simulink model "Main"  (R2022b)
settings: Solver=VariableStepAuto  StartTime=0.0  StopTime=3.0  RelTol=1e-3
undefined symbols (not defined in the file): a, dc, I, K, L, m
settings Model: Creator=pagli  LastModifiedBy=pagli
settings SolverCC: ZeroCrossControl=DisableAll

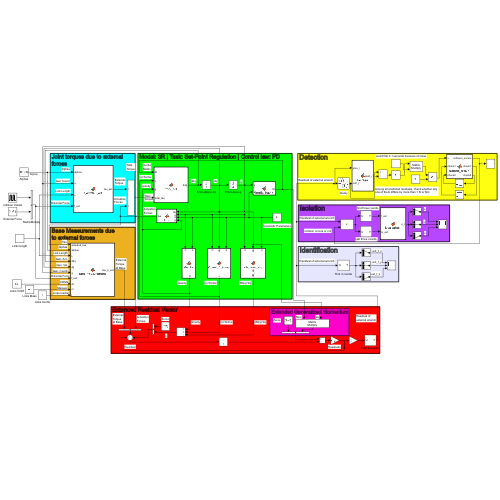
[thumbnail: Simulink's stored preview of the top-level diagram]
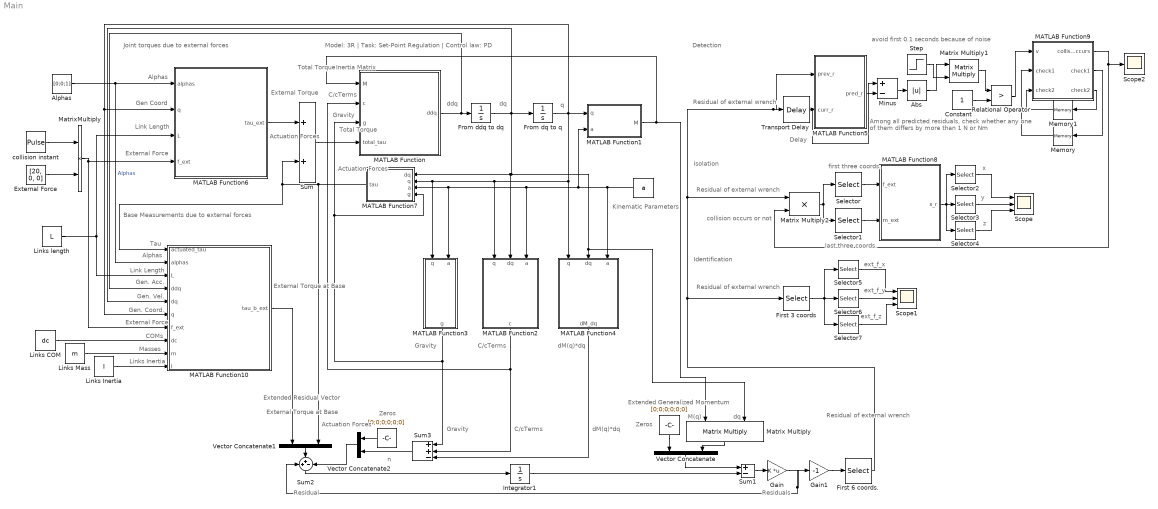
== system Main ==
  note: ext_f_x
  note: z
  note: y
  note: x
  note: Among all predicted residuals, check whether any
      | one of them differs by more than 1 N or Nm
  note: avoid first 0.1 seconds because of noise
  note: Delay
  note: first three coords.
  note: collision occurs or not
  note: Extended Generalized Momentum
  note: Identification
  note: Tau
  note: Alphas
  note: Isolation
  note: Detection
  note: n
  note: Residual
  note: External
      | Torque
      | at Base
  note: Links Inertia
  note: Masses
  note: COMs
  note: Gen. Coord.
  note: Gen. Vel.
  note: Gen. Acc.
  note: dM(q)*dq
  note: Kinematic Parameters
  note: q
  note: dq
  note: ddq
  note: Actuation
      | Forces
  note: Gravity
  note: C/cTerms
  note: Inertia
      | Matrix
  note: External
      | Torque
  note: External Force
  note: Link Length
  note: Gen Coord
  note: Alphas
  note: Zeros
  note: M(q)
  note: dq
  note: Joint torques due to external
      | forces
  note: Base Measurements due
      | to external forces
  note: Model: 3R | Task: Set-Point Regulation | Control law: PD
  note: Extended Residual Vector
  note: Zeros
  note: Total
      | Torque
  note: Gravity
  note: C/cTerms
  note: Link Length
  note: External Force
  note: External
      | Torque
      | at Base
  note: Actuation
      | Forces
  note: Gravity
  note: C/cTerms
  note: dM(q)*dq
  note: Residuals
  note: Residual of external wrench
  note: Residual of external wrench
  note: last three coords.
  note: Actuation
      | Forces
  note: Total
      | Torque
  note: Residual of
      | external wrench
  note: Residual of external wrench
  note: ext_f_y
  note: ext_f_z
  " " : Constant  Value=[0;0;0;0;0;0]
  "  " : Constant  Value=[0;0;0;0;0;0]
  "   " : Constant  Value=a
  Abs : Abs  SaturateOnIntegerOverflow=off
  Alphas : Constant  Value=[0;0;1]  OutDataTypeStr=double
  Constant : Constant
  External Force : Constant  Value=[20, 0, 0]
  First 3 coords : Selector  InputPortWidth=6  IndexOptions=Index vector (dialog)  Indices=[1 2 3]  OutputSizes=1
  First 6 coords. : Selector  InputPortWidth=9  IndexOptions=Index vector (dialog)  Indices=[1 2 3 4 5 6]  OutputSizes=1
  From ddq to dq : Integrator  InitialCondition=[0;0;0]
  From dq to q : Integrator  InitialCondition=[0; pi/2; 0]
  Gain : Gain  Gain=K  Multiplication=Matrix(K*u)
  Gain1 : Gain  Gain=-1
  Integrator1 : Integrator  InitialCondition=[0;0;0;0;0;0;0;0;0]
  Links COM : Constant  Value=dc
  Links Inertia : Constant  Value=I
  Links Mass : Constant  Value=m
  Links length : Constant  Value=L
  MATLAB Function : MATLAB Function  TreatAsAtomicUnit=on
  MATLAB Function1 : MATLAB Function  TreatAsAtomicUnit=on
  MATLAB Function10 : MATLAB Function  TreatAsAtomicUnit=on
  MATLAB Function2 : MATLAB Function  TreatAsAtomicUnit=on
  MATLAB Function3 : MATLAB Function  TreatAsAtomicUnit=on
  MATLAB Function4 : MATLAB Function  TreatAsAtomicUnit=on
  MATLAB Function5 : MATLAB Function  TreatAsAtomicUnit=on
  MATLAB Function6 : MATLAB Function  TreatAsAtomicUnit=on
  MATLAB Function7 : MATLAB Function  TreatAsAtomicUnit=on
  MATLAB Function8 : MATLAB Function  TreatAsAtomicUnit=on
  MATLAB Function9 : MATLAB Function  TreatAsAtomicUnit=on
  Matrix Multiply : Product  Multiplication=Matrix(*)
  Matrix Multiply1 : Product  Multiplication=Matrix(*)
  Matrix Multiply2 : Product
  MatrixMultiply : Product
  Memory : Memory  InitialCondition=0.0
  Memory1 : Memory  InitialCondition=0.0
  Minus : Sum  Inputs=+-
  Relational Operator : RelationalOperator  Operator=>  OutDataTypeStr=boolean  RndMeth=Simplest  InputSameDT=off
  Scope : Scope  NumInputPorts=3
  Scope1 : Scope  NumInputPorts=3
  Scope2 : Scope
  Selector : Selector  InputPortWidth=6  IndexOptions=Index vector (dialog)  Indices=[1 2 3]  OutputSizes=1
  Selector1 : Selector  InputPortWidth=6  IndexOptions=Index vector (dialog)  Indices=[4 5 6]  OutputSizes=1
  Selector2 : Selector  InputPortWidth=3  IndexOptions=Index vector (dialog)  Indices=[1]  OutputSizes=1
  Selector3 : Selector  InputPortWidth=3  IndexOptions=Index vector (dialog)  Indices=[2]  OutputSizes=1
  Selector4 : Selector  InputPortWidth=3  IndexOptions=Index vector (dialog)  Indices=[3]  OutputSizes=1
  Selector5 : Selector  InputPortWidth=3  IndexOptions=Index vector (dialog)  Indices=[1]  OutputSizes=1
  Selector6 : Selector  InputPortWidth=3  IndexOptions=Index vector (dialog)  Indices=[2]  OutputSizes=1
  Selector7 : Selector  InputPortWidth=3  IndexOptions=Index vector (dialog)  Indices=[3]  OutputSizes=1
  Step : Step  Time=0.5  SampleTime=0
  Sum : Sum
  Sum1 : Sum  Inputs=+-
  Sum2 : Sum  Inputs=++-
  Sum3 : Sum  Inputs=++-
  Transport Delay : TransportDelay  DelayTime=0.005  BufferSize=4096
  Vector Concatenate : Concatenate
  Vector Concatenate1 : Concatenate
  Vector Concatenate2 : Concatenate
  collision instant : DiscretePulseGenerator  PulseType=Time based  Period=5  PhaseDelay=1.8
  wires:
  MATLAB Function/1(ddq) -> MATLAB Function10/4(ddq), From ddq to dq/1
  From ddq to dq/1 -> MATLAB Function2/2(dq), MATLAB Function7/1(dq), MATLAB Function4/2(dq), Matrix Multiply/2, MATLAB Function10/5(dq), From dq to q/1
  From dq to q/1 -> MATLAB Function6/2(q), MATLAB Function10/6(q), MATLAB Function4/1(q), MATLAB Function3/1(q), MATLAB Function7/2(q), MATLAB Function2/1(q), MATLAB Function1/1(q)
  "   "/1 -> MATLAB Function4/3(a), MATLAB Function1/2(a), MATLAB Function2/3(a), MATLAB Function3/2(a), MATLAB Function7/3(a)
  MATLAB Function6/1(tau_ext) -> Sum/1
  MATLAB Function7/1(tau) -> MATLAB Function10/1(actuated_tau), Sum/2, Vector Concatenate1/2
  Sum/1 -> MATLAB Function/4(total_tau)
  MATLAB Function3/1(g) -> Sum3/1, MATLAB Function7/4(g), MATLAB Function/3(g)
  MATLAB Function2/1(c) -> MATLAB Function/2(c), Sum3/2
  MATLAB Function1/1(M) -> Matrix Multiply/1, MATLAB Function/1(M)
  " "/1 -> Vector Concatenate/1
  MATLAB Function4/1(dM_dq) -> Sum3/3
  Sum3/1 -> Vector Concatenate2/2
  "  "/1 -> Vector Concatenate2/1
  Vector Concatenate1/1 -> Sum2/2
  MATLAB Function10/1(tau_b_ext) -> Vector Concatenate1/1
  Sum2/1 -> Integrator1/1
  Sum1/1 -> Gain/1
  Integrator1/1 -> Sum1/2
  Vector Concatenate/1 -> Sum1/1
  collision instant/1 -> MatrixMultiply/1
  External Force/1 -> MatrixMultiply/2
  Alphas/1 -> MATLAB Function6/1(alphas), MATLAB Function10/2(alphas)  "Alphas"
  Links length/1 -> MATLAB Function6/3(L), MATLAB Function10/3(L)
  MatrixMultiply/1 -> MATLAB Function6/4(f_ext), MATLAB Function10/7(f_ext)
  Links COM/1 -> MATLAB Function10/8(dc)
  Links Mass/1 -> MATLAB Function10/9(m)
  Links Inertia/1 -> MATLAB Function10/10(I)
  Matrix Multiply/1 -> Vector Concatenate/2
  Vector Concatenate2/1 -> Sum2/3
  Gain/1 -> Sum2/1, Gain1/1
  Transport Delay/1 -> Minus/1, MATLAB Function5/2(curr_r)
  MATLAB Function5/1(pred_r) -> Minus/2
  Constant/1 -> Relational Operator/2
  Minus/1 -> Abs/1
  Matrix Multiply1/1 -> Relational Operator/1
  Abs/1 -> Matrix Multiply1/1
  Step/1 -> Matrix Multiply1/2
  Relational Operator/1 -> MATLAB Function9/1(v)
  Selector/1 -> MATLAB Function8/1(f_ext)
  Selector1/1 -> MATLAB Function8/2(m_ext)
  MATLAB Function8/1(x_r) -> Selector4/1, Selector2/1, Selector3/1
  Matrix Multiply2/1 -> Selector/1, Selector1/1
  MATLAB Function9/1(collision_occurs) -> Scope2/1, Matrix Multiply2/2
  First 6 coords./1 -> MATLAB Function5/1(prev_r), Transport Delay/1, Matrix Multiply2/1, First 3 coords/1
  Gain1/1 -> First 6 coords./1
  MATLAB Function9/2(check1) -> Memory/1
  Memory/1 -> MATLAB Function9/2("check1 ")
  Memory1/1 -> MATLAB Function9/3("check2 ")
  MATLAB Function9/3(check2) -> Memory1/1
  Selector2/1 -> Scope/1
  Selector3/1 -> Scope/2
  Selector4/1 -> Scope/3
  Selector7/1 -> Scope1/3
  First 3 coords/1 -> Selector5/1, Selector7/1, Selector6/1
  Selector5/1 -> Scope1/1
  Selector6/1 -> Scope1/2

== matlab function Main/MATLAB Function10 ==
  data: actuated_tau input; alphas input; L input; ddq input; dq input; q input; f_ext input; tau_b_ext output; dc input; m input; I input
function tau_b_ext = base_measurements(actuated_tau, alphas, L, ddq, dq, q, f_ext, dc, m, I)
    alpha1 = alphas(1); alpha2 = alphas(2); alpha3 = alphas(3); 
    q1 = q(1); q2 = q(2); q3 = q(3);
    
    R = zeros(3, 3, 3);
    R(:, :, 1) = [cos(q1), 0,  sin(q1);
                  sin(q1), 0, -cos(q1);
                        0, 1,        0];
    R(:, :, 2) = [cos(q2), -sin(q2), 0;
                  sin(q2),  cos(q2), 0;
                        0,        0, 1];
    R(:, :, 3) = [cos(q3), -sin(q3), 0;
                  sin(q3),  cos(q3), 0;
                        0,        0, 1];

    omega = zeros(3, 3);
    d_omega = zeros(3, 3);
    iMinus1_omega_iMinus1 = [0;0;0];
    iMinus1_d_omega_iMinus1 = [0;0;0];
    for i = 1 : 1 : 3
        iMinus1_R_i = R(:, :, i);

        i_omega_i = (iMinus1_R_i') * (iMinus1_omega_iMinus1 + dq(i)*[0;0;1]);
        omega(:, i) = i_omega_i;

        i_d_omega_i = (iMinus1_R_i') * (iMinus1_d_omega_iMinus1 + ddq(i)*[0;0;1] + cross(dq(i)*iMinus1_omega_iMinus1, [0;0;1]));
        d_omega(:, i) = i_d_omega_i;

        iMinus1_omega_iMinus1 = i_omega_i;
        iMinus1_d_omega_iMinus1 = i_d_omega_i;
    end

    a = zeros(3, 3);
    ac = zeros(3, 3);
    iMinus1_a_iMinus1 = [0;0;0];
    r = zeros(3,3);
    r(:, 1) = [0; -L(1); 0];
    r(:, 2) = [-L(2); 0; 0];
    r(:, 3) = [-L(3); 0; 0];
    rc = zeros(3,3);
    rc(:, 1) = [          0; dc(1); 0];
    rc(:, 2) = [dc(2);           0; 0];
    rc(:, 3) = [dc(3);           0; 0];
%     for i = 1 : 1 : 3
%         iMinus1_R_i = R(:, :, i);
% 
%         i_a_i = (iMinus1_R_i') * iMinus1_a_iMinus1 + cross(d_omega(:, i), r(:, i)) + cross(omega(:, i), cross(omega(:, i), r(:, i)));
%         a(:, i) = i_a_i;
% 
%         i_ac_i = i_a_i + cross(d_omega(:, i), rc(:, i)) + cross(omega(:, i), cross(omega(:, i), rc(:, i)));
%         ac(:, i) = i_ac_i;
% 
%         iMinus1_a_iMinus1 = i_a_i;
%     end

    f = zeros(3, 3);
    tau = zeros(3, 3);
    g = zeros(3, 3);
    g(:, 1) = R(:, :, 1)'*[0;0;9.81];
    g(:, 2) = R(:, :, 2)'*(R(:, :, 1)'*[0;0;9.81]);
    g(:, 3) = R(:, :, 3)'*(R(:, :, 2)'*(R(:, :, 1)'*[0;0;9.81]));
    iPlus1_tau_iPlus1 = [0;0;0];
    iPlus1_f_iPlus1 = [0;0;0];
    iPlus1_f_iPlus1 = R(:, :, 3)'*(R(:, :, 2)'*(R(:, :, 1)'*f_ext));
    i_R_iPlus1 = eye(3);
    for i = 3 : -1 : 1
%         if alpha3 > 0
%             iPlus1_f_iPlus1 = R(:, :, 3)'*(R(:, :, 2)'*(R(:, :, 1)'*f_ext));
%         elseif alpha2 > 0
%             iPlus1_f_iPlus1 = iPlus1_f_iPlus1 + R(:, :, 2)'*(R(:, :, 1)'*f_ext);
%         elseif alpha1 > 0
%             iPlus1_f_iPlus1 = iPlus1_f_iPlus1 + R(:, :, 1)'*f_ext;
%         end
        i_f_i = i_R_iPlus1*iPlus1_f_iPlus1+ m(i)*(ac(:, i));
        f(:, i) = i_f_i;

        i_tau_i = i_R_iPlus1*iPlus1_tau_iPlus1 + cross(i_R_iPlus1*iPlus1_f_iPlus1, rc(:, i)) - cross(i_f_i, r(:, i)+rc(:, i)); %+ I(:,:,i)*d_omega(:, i) + cross(omega(:, i), I(:,:,i)*omega(:, i));
        tau(:, i) = i_tau_i;

        iPlus1_f_iPlus1 = i_f_i;
        iPlus1_tau_iPlus1 = i_tau_i;
        i_R_iPlus1 = R(:, :, i);
    end

    tau_0 = R(:, :, 1)*tau(:, 1);
    f_0 = R(:, :, 1)*f(:, 1);
    tau_b_ext = [f_0; -tau_0];

== matlab function Main/MATLAB Function1 ==
  data: q input; M output; a input
function M = Inertia_Matrix(q, a)
    % joint angles
    q1 = q(1); q2 = q(2); q3 = q(3);
    % Constant Element of Inertia Matrix
    a1 = a(1); a2 = a(2); a3 = a(3); a4 = a(4);
    a5 = a(5); a6 = a(6);
    % Inertia Matrix Components
    m11 = a1 + a4*cos(q3) + a4*cos(2*q2 + q3) + a3*cos(q2 + q3)^2 + a2*cos(q2)^2;
    m12 = 0;
    m21 = 0;
    m13 = 0;
    m31 = 0;
    m22 = a5 + 2*a4*cos(q3);
    m23 = a6 + a4*cos(q3);
    m32 = a6 + a4*cos(q3);
    m33 = a6;
    % Inertia Matrix
    M = [m11, m12, m13;
         m21, m22, m23;
         m31, m32, m33];

== matlab function Main/MATLAB Function ==
  data: M input; c input; g input; total_tau input; ddq output
function ddq = robot_3R(M, c, g, total_tau)
    % considering the dynamic model M*ddq + c + g = total_tau = tau + tau_ext    
    persistent x

    if isempty(x)
        x = 1;
    end

    if (x==1)
        ddq = M\(total_tau - c - g);
    else
        ddq = [0;0;0];
    end

== matlab function Main/MATLAB Function2 ==
  data: q input; c output; dq input; a input
function c = C_and_C_terms(q, dq, a)
    % joint angles
    q2 = q(2); q3 = q(3);
    % joint velocites
    dq1 = dq(1); dq2 = dq(2); dq3 = dq(3);
    % Constant Element of Inertia Matrix
    a2 = a(2); a3 = a(3); a4 = a(4);
    % first component of Coriolis/Centrifugal terms
    c1 = - dq1*(dq2*(a4*sin(2*q2 + q3) + a3*cos(q2 + q3)*sin(q2 + q3) + a2*cos(q2)*sin(q2)) + dq3*((a4*sin(q3))/2 + (a4*sin(2*q2 + q3))/2 + a3*cos(q2 + q3)*sin(q2 + q3))) - dq1*dq3*((a4*sin(q3))/2 + (a4*sin(2*q2 + q3))/2 + a3*cos(q2 + q3)*sin(q2 + q3)) - dq1*dq2*(a4*sin(2*q2 + q3) + a3*cos(q2 + q3)*sin(q2 + q3) + a2*cos(q2)*sin(q2));
    % second component of Coriolis/Centrifugal terms
    c2 = (a4*sin(2*q2 + q3) + a3*cos(q2 + q3)*sin(q2 + q3) + a2*cos(q2)*sin(q2))*dq1^2 - dq3*(a4*dq2*sin(q3) + a4*dq3*sin(q3)) - a4*dq2*dq3*sin(q3);
    % third component of Coriolis/Centrifugal terms
    c3 = ((a4*sin(q3))/2 + (a4*sin(2*q2 + q3))/2 + a3*cos(q2 + q3)*sin(q2 + q3))*dq1^2 + a4*sin(q3)*dq2^2;
    % Coriolis/Centrifugal terms
    c = [c1; c2; c3];

== matlab function Main/MATLAB Function3 ==
  data: q input; g output; a input
function g = Gravity(q, a)
    % joint angle
    q2 = q(2); q3 = q(3);
    % Constant Element of Inertia Matrix
    a7 = a(7); a8 = a(8);
    % first component of gravitational term
    g1 = 0;
    % second component of gravitational term
    g2 = a8*cos(q2 + q3) + a7*cos(q2);
    % third component of gravitational term
    g3 = a8*cos(q2 + q3);
    % Gravitational term of dynamic model
    g = [g1; g2; g3];

== matlab function Main/MATLAB Function4 ==
  data: q input; dM_dq output; dq input; a input
function dM_dq = dM_times_dq(q, dq, a)
    % joint angles
    q2 = q(2); q3 = q(3);
    % joint velocities
    dq2 = dq(2); dq3 = dq(3);
    % Constant Element of Inertia Matrix
    a2 = a(2); a3 = a(3); a4 = a(4);
    % Components of Inertia Matrix Derivative
    dm11 = - dq2*(2*a4*sin(2*q2 + q3) + 2*a3*cos(q2 + q3)*sin(q2 + q3) + 2*a2*cos(q2)*sin(q2)) - dq3*(a4*sin(q3) + a4*sin(2*q2 + q3) + 2*a3*cos(q2 + q3)*sin(q2 + q3));
    dm12 = 0;
    dm21 = 0;
    dm13 = 0;
    dm31 = 0;
    dm22 = -2*a4*dq3*sin(q3);
    dm23 = -a4*dq3*sin(q3);
    dm32 = -a4*dq3*sin(q3);
    dm33 = 0;
    % Inertia Matrix Derivative
    dM = [dm11, dm12, dm13;
          dm21, dm22, dm23;
          dm31, dm32, dm33];
    
    dM_dq = dM * dq;

== matlab function Main/MATLAB Function5 ==
  data: prev_r input; curr_r input; pred_r output
function pred_r = average(prev_r, curr_r)
    %equation of line segment between two points
    pred_r = (curr_r + prev_r)/2;

== matlab function Main/MATLAB Function6 ==
  data: alphas input; q input; L input; f_ext input; tau_ext output
function tau_ext = f_ext2tau_ext(alphas, q, L, f_ext)
    % joint angles
    q1 = q(1); q2 = q(2); q3 = q(3); 
    % links length
    L2 = L(2); L3 = L(3);
    
    alpha2 = alphas(2); alpha3 = alphas(3);
    if alpha3 > 0
        aL2 = 1; aL3 = alpha3*L3;
    elseif alpha2 > 0
        aL2 = alpha2*L2; aL3 = 0;
    else
        aL2 = 0; aL3 = 0;
    end
    
    % first row of (contact) Jacobian
    J1 = [-sin(q1)*(aL3*cos(q2+q3)+aL2*cos(q2)), -cos(q1)*(aL3*sin(q2+q3)+aL2*sin(q2)), -cos(q1)*aL3*sin(q2+q3)];
    % second row of (contact) Jacobian
    J2 = [ cos(q1)*(aL3*cos(q2+q3)+aL2*cos(q2)), -sin(q1)*(aL3*sin(q2+q3)+aL2*sin(q2)), -sin(q1)*aL3*sin(q2+q3)];
    % third row if (contact) Jacobian
    J3 = [                                    0,            aL3*cos(q2+q3)+aL2*cos(q2),          aL3*cos(q2+q3)];
    % (contact) Jacobian
    J = [J1; J2; J3];
    % torques exerted at joints
    tau_ext = J'*f_ext;

== matlab function Main/MATLAB Function7 ==
  data: dq input; tau output; q input; a input; g input
function tau = PD(dq, q, a, g)
    a7 = a(7); a8 = a(8);
    Kp = eye(3)*10;
    Kd = eye(3)*10;
    qd = [0;pi/2;0];
    tau = Kp*(qd - q) - Kd*dq + g;

== matlab function Main/MATLAB Function8 ==
  data: f_ext input; x_r output; m_ext input
function x_r = localization(f_ext, m_ext)
    S = [ 0       , -f_ext(3),  f_ext(2);
          f_ext(3),         0, -f_ext(1);
         -f_ext(2),  f_ext(1),    0];
    pinv_S = -pinv(S);
    x_r = pinv_S*m_ext;

== matlab function Main/MATLAB Function9 ==
  data: v input; collision_occurs output double size=1 [0..]; check1 output; check1 input; check2 input; check2 output
function [collision_occurs, check1, check2] = collision_check(v, check1, check2)
    if (v(1) || v(2) || v(3) || v(4) || v(5) || v(6)) && check1 == 0.0
        collision_occurs = 1.0;
        check1 = 1.0;
        check2 = 0.0;
    elseif (v(1) || v(2) || v(3) || v(4) || v(5) || v(6)) && check1 == 1.0 && check2 == 0.0
        collision_occurs = 1.0;
        check1 = 1.0;
        check2 = 0.0;
    elseif not(v(1) || v(2) || v(3) || v(4) || v(5) || v(6)) && check1 == 1.0 && check2 == 0.0
        collision_occurs = 0.0;
        check1 = 1.0;
        check2 = 1.0;
    elseif not(v(1) || v(2) || v(3) || v(4) || v(5) || v(6)) && check1 == 0.0 && check2 == 0.0
        collision_occurs = 0.0;
        check1 = 0.0;
        check2 = 0.0;
    else
        collision_occurs = 0.0;
        check1 = 1.0;
        check2 = 1.0;
    end
